simulink model "EngineModel_scaled_15_7_2016_with_new_maps"  (R2021a)
settings: Solver=ode4  StartTime=0.0  StopTime=30  FixedStep=0.2  RelTol=1e-3  EnableMultiTasking=on
values from neighbouring files (symbols this model uses):
  Fanmap_2 = [1 1 1 1 1 1 1 1 1 1 275.724 325.4224 ... (330 elements, 10x3x11)]    [enginemaps2.mat]
  HPCompmap_2 = [1 1 1 1 1 1 1 1 1 1 32.390865 37.6623195 ... (330 elements, 10x3x11)]    [enginemaps2.mat]
  HPTurbinemap_2 = [0.24979968 0.24979968 0.24979968 0.24979968 0.24979968 0.24979968 0.24979968 0.24979968 0.24979968 0.24979968 0.004250667 0.005047667 ... (330 elements, 10x3x11)]    [enginemaps2.mat]
  LPCompmap_2 = [1 1 1 1 1 1 1 1 1 1 34.17260994 40.23277722 ... (330 elements, 10x3x11)]    [enginemaps2.mat]
  LPTurbinemap_2 = [0.665969797 0.665969797 0.665969797 0.665969797 0.665969797 0.665969797 0.665969797 0.665969797 0.00912 0.013173333 0.015706667 0.01672 ... (264 elements, 8x3x11)]    [enginemaps2.mat]
undefined symbols (not defined in the file or in its folder): Adiabatic_compression_fan, Adiabatic_compression_HPC, Adiabatic_compression_LPC, coldnozzle, compression_ram, cond_f2, D, datatables, hotnozzle, HPT1, if_Nth, if_Ntl, if_Z, LPT, performance1, thermo_combustor, turbo
libraries: dspmtrx3 x10, aerolibatmos2 x8, dspsigattribs x3, dspsolvers x2, dspfactors x1
(part 2 of 13)

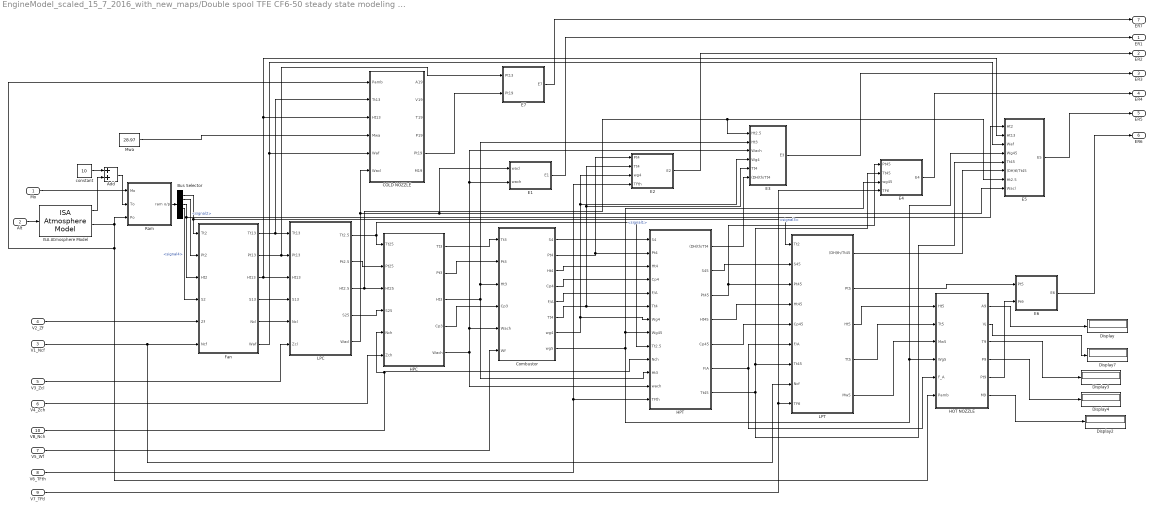
== system EngineModel_scaled_15_7_2016_with_new_maps/Double spool TFE CF6-50 steady state modeling (BOING 747-200)/Error Due to Vs/Error Due To Dv5 ==
  Mo : Inport
  Alt : Inport  Port=2
  V1_Ncf : Inport  Port=3
  V2_Zf : Inport  Port=4
  V3_Zcl : Inport  Port=5
  V4_Zch : Inport  Port=6
  V5_Wf : Inport  Port=7
  V6_TFth : Inport  Port=8
  V7_TFtl : Inport  Port=9
  VB_Nch : Inport  Port=10
  Add : Sum
  Bus Selector : BusSelector  OutputSignals=signal1,signal2,signal3,signal4,signal5
  COLD NOZZLE : Subsystem
  Combustor : Subsystem
  Display{,2..4,7} (5 alike) : Display
  E1 : Subsystem
  E2 : Subsystem
  E3 : Subsystem
  E4 : Subsystem
  E5 : Subsystem
  E6 : Subsystem
  E7 : Subsystem
  Fan : Subsystem
  HOT NOZZLE : Subsystem
  HPC : Subsystem
  HPT : Subsystem
  ISA Atmosphere Model : aerolibatmos2/ISA Atmosphere Model  custom=on  g=9.81  gamma=1.4  R=287  L=0.0065  h_trop=11000  h_strat=20000  rho0=1.225  P0=101325  T0=288  h0=0
  LPC : Subsystem
  LPT : Subsystem
  Mwa : Constant  Value=28.97
  Ram : Subsystem
  constant : Constant  Value=10
  ER1 : Outport
  ER2 : Outport  Port=2
  ER3 : Outport  Port=3
  ER4 : Outport  Port=4
  ER5 : Outport  Port=5
  ER6 : Outport  Port=6
  ER7 : Outport  Port=7
  wires:
  Alt/1 -> ISA Atmosphere Model/1
  Mo/1 -> Ram/1(Mo)
  ISA Atmosphere Model/1 -> Add/2
  Ram/1(ram o/p) -> Bus Selector/1
  ISA Atmosphere Model/3 -> Ram/3(Po), COLD NOZZLE/1(Pamb), HOT NOZZLE/6(Pamb)
  constant/1 -> Add/1
  Add/1 -> Ram/2(To)
  Bus Selector/1 -> Fan/1(Tt2), LPT/1(Tt2)  "<signal1>"
  Bus Selector/2 -> Fan/2(Pt2)  "<signal2>"
  Fan/1(Tt13) -> LPC/1(Tt13), COLD NOZZLE/2(Tt13)
  Fan/2(Pt13) -> E7/1(Pt13), LPC/2(Pt13)
  LPC/1(Tt2.5) -> HPC/1(Tt25), HPT/9(Tt2.5)
  LPC/2(Pt2.5) -> HPC/2(Pt25)
  HPC/1(Tt3) -> Combustor/1(Tt3)
  HPC/2(Pt3) -> Combustor/2(Pt3)
  HPC/3(Ht3) -> Combustor/3(Ht3), E3/2(Ht3), HPT/11(Ht3)
  Combustor/2(Pt4) -> E2/1(Pt4), HPT/2(Pt4)
  Combustor/4(Cp4) -> HPT/4(Cp4)
  Combustor/5(F/A) -> HPT/5(F/A)
  Combustor/6(Tt4) -> E2/2(Tt4), E3/5(Tt4), HPT/6(Tt4)
  LPT/3(Ht5) -> HOT NOZZLE/1(Ht5)
  LPT/4(Tt5) -> HOT NOZZLE/2(Tt5)
  V2_Zf/1 -> Fan/5(Zf)
  V1_Ncf/1 -> LPT/8(Ncf), Fan/6(Ncf)
  V3_Zcl/1 -> LPC/6(Zcl)
  V4_Zch/1 -> HPC/6(Zch)
  VB_Nch/1 -> HPT/10(Nch), HPC/5(Nch)
  V5_Wf/1 -> Combustor/6(Wf)
  V6_TFth/1 -> E2/4(TFth), HPT/13(TFth)
  Combustor/7(wg4) -> E2/3(wg4), E3/4(Wg4), HPT/7(Wg4)
  LPT/5(Mw5) -> HOT NOZZLE/3(Mw5)
  Fan/3(Ht13) -> COLD NOZZLE/3(Ht13), E5/2(Ht13), LPC/3(Ht13)
  Mwa/1 -> COLD NOZZLE/4(Mwa)
  Fan/6(Waf) -> E5/3(Waf), COLD NOZZLE/5(Waf)
  LPC/5(Wacl) -> COLD NOZZLE/6(Wacl), E1/1(wacl), E5/8(Wacl)
  COLD NOZZLE/5(Pt19) -> E7/2(Pt19)
  LPC/3(Ht2.5) -> HPC/3(Ht25), E3/1(Ht2.5), E5/7(Ht2.5)
  LPT/2(Pt5) -> E6/1(Pt5)
  HOT NOZZLE/5(Pt9) -> E6/2(Pt9)
  LPT/1((DH)th/Tt45) -> E5/6((DH)tl/Tt45)
  Combustor/8(wg5) -> E4/3(wg45), HPT/8(Wg45), E5/4(Wg45), HOT NOZZLE/4(Wg5)
  Combustor/3(Ht4) -> HPT/3(Ht4)
  Combustor/1(S4) -> HPT/1(S4)
  HOT NOZZLE/1(A9) -> Display/1
  HOT NOZZLE/2(Vj) -> Display7/1
  HOT NOZZLE/3(T9) -> Display3/1
  HOT NOZZLE/4(P9) -> Display4/1
  HOT NOZZLE/6(M9) -> Display2/1
  Bus Selector/3 -> Fan/3(Ht2), E5/1(Ht2)  "<signal3>"
  Bus Selector/4 -> Fan/4(S2)  "<signal4>"
  Fan/5(Ncl) -> LPC/5(Ncl)
  Fan/4(S13) -> LPC/4(S13)
  LPC/4(S25) -> HPC/4(S25)
  HPC/5(Wach) -> Combustor/5(Wach), E3/3(Wach), E1/2(wach), HPT/12(wach)
  HPT/2(S45) -> LPT/2(S45)
  HPT/3(Pt45) -> E4/1(Pt45), LPT/3(Pt45)
  HPT/4(Ht45) -> LPT/4(Ht45)
  HPT/5(Cp45) -> LPT/5(Cp45)
  HPT/7(Tt45) -> LPT/7(Tt45), E4/2(Tt45), E5/5(Tt45)
  HPT/6(F\A) -> LPT/6(F/A), HOT NOZZLE/5(F_A)
  V7_TFtl/1 -> LPT/9(TFtl), E4/4(TFtl)
  HPT/1((DH)th/Tt4) -> E3/6((DH)th/Tt4)
  E6/1(E6) -> ER6/1
  E5/1(E5) -> ER5/1
  E4/1(E4) -> ER4/1
  E3/1(E3) -> ER3/1
  E2/1(E2) -> ER2/1
  E1/1(E1) -> ER1/1
  E7/1(E7) -> ER7/1
  HPC/4(Cp3) -> Combustor/4(Cp3)

== system EngineModel_scaled_15_7_2016_with_new_maps/Double spool TFE CF6-50 steady state modeling (BOING 747-200)/Error Due to Vs/Error Due To Dv6 ==
  Mo : Inport
  Alt : Inport  Port=2
  V1_Ncf : Inport  Port=3
  V2_Zf : Inport  Port=4
  V3_Zcl : Inport  Port=5
  V4_Zch : Inport  Port=6
  V5_Wf : Inport  Port=7
  V6_TFth : Inport  Port=8
  V7_TFtl : Inport  Port=9
  VB_Nch : Inport  Port=10
  Add : Sum
  Bus Selector : BusSelector  OutputSignals=signal1,signal2,signal3,signal4,signal5
  COLD NOZZLE : Subsystem
  Combustor : Subsystem
  Display{,2..4,7} (5 alike) : Display
  E1 : Subsystem
  E2 : Subsystem
  E3 : Subsystem
  E4 : Subsystem
  E5 : Subsystem
  E6 : Subsystem
  E7 : Subsystem
  Fan : Subsystem
  HOT NOZZLE : Subsystem
  HPC : Subsystem
  HPT : Subsystem
  ISA Atmosphere Model : aerolibatmos2/ISA Atmosphere Model  custom=on  g=9.81  gamma=1.4  R=287  L=0.0065  h_trop=11000  h_strat=20000  rho0=1.225  P0=101325  T0=288  h0=0
  LPC : Subsystem
  LPT : Subsystem
  Mwa : Constant  Value=28.97
  Ram : Subsystem
  constant : Constant  Value=10
  ER1 : Outport
  ER2 : Outport  Port=2
  ER3 : Outport  Port=3
  ER4 : Outport  Port=4
  ER5 : Outport  Port=5
  ER6 : Outport  Port=6
  ER7 : Outport  Port=7
  wires:
  HPC/4(Cp3) -> Combustor/4(Cp3)
  E7/1(E7) -> ER7/1
  E1/1(E1) -> ER1/1
  E2/1(E2) -> ER2/1
  E3/1(E3) -> ER3/1
  E4/1(E4) -> ER4/1
  E5/1(E5) -> ER5/1
  E6/1(E6) -> ER6/1
  HPT/1((DH)th/Tt4) -> E3/6((DH)th/Tt4)
  V7_TFtl/1 -> E4/4(TFtl), LPT/9(TFtl)
  HPT/6(F\A) -> HOT NOZZLE/5(F_A), LPT/6(F/A)
  HPT/7(Tt45) -> E5/5(Tt45), E4/2(Tt45), LPT/7(Tt45)
  HPT/5(Cp45) -> LPT/5(Cp45)
  HPT/4(Ht45) -> LPT/4(Ht45)
  HPT/3(Pt45) -> LPT/3(Pt45), E4/1(Pt45)
  HPT/2(S45) -> LPT/2(S45)
  HPC/5(Wach) -> HPT/12(wach), E1/2(wach), E3/3(Wach), Combustor/5(Wach)
  LPC/4(S25) -> HPC/4(S25)
  Fan/4(S13) -> LPC/4(S13)
  Fan/5(Ncl) -> LPC/5(Ncl)
  Bus Selector/4 -> Fan/4(S2)  "<signal4>"
  Bus Selector/3 -> E5/1(Ht2), Fan/3(Ht2)  "<signal3>"
  HOT NOZZLE/6(M9) -> Display2/1
  HOT NOZZLE/4(P9) -> Display4/1
  HOT NOZZLE/3(T9) -> Display3/1
  HOT NOZZLE/2(Vj) -> Display7/1
  HOT NOZZLE/1(A9) -> Display/1
  Combustor/1(S4) -> HPT/1(S4)
  Combustor/3(Ht4) -> HPT/3(Ht4)
  Combustor/8(wg5) -> HOT NOZZLE/4(Wg5), E5/4(Wg45), HPT/8(Wg45), E4/3(wg45)
  LPT/1((DH)th/Tt45) -> E5/6((DH)tl/Tt45)
  HOT NOZZLE/5(Pt9) -> E6/2(Pt9)
  LPT/2(Pt5) -> E6/1(Pt5)
  LPC/3(Ht2.5) -> E5/7(Ht2.5), E3/1(Ht2.5), HPC/3(Ht25)
  COLD NOZZLE/5(Pt19) -> E7/2(Pt19)
  LPC/5(Wacl) -> E5/8(Wacl), E1/1(wacl), COLD NOZZLE/6(Wacl)
  Fan/6(Waf) -> COLD NOZZLE/5(Waf), E5/3(Waf)
  Mwa/1 -> COLD NOZZLE/4(Mwa)
  Fan/3(Ht13) -> LPC/3(Ht13), E5/2(Ht13), COLD NOZZLE/3(Ht13)
  LPT/5(Mw5) -> HOT NOZZLE/3(Mw5)
  Combustor/7(wg4) -> HPT/7(Wg4), E3/4(Wg4), E2/3(wg4)
  V6_TFth/1 -> HPT/13(TFth), E2/4(TFth)
  V5_Wf/1 -> Combustor/6(Wf)
  VB_Nch/1 -> HPC/5(Nch), HPT/10(Nch)
  V4_Zch/1 -> HPC/6(Zch)
  V3_Zcl/1 -> LPC/6(Zcl)
  V1_Ncf/1 -> Fan/6(Ncf), LPT/8(Ncf)
  V2_Zf/1 -> Fan/5(Zf)
  LPT/4(Tt5) -> HOT NOZZLE/2(Tt5)
  LPT/3(Ht5) -> HOT NOZZLE/1(Ht5)
  Combustor/6(Tt4) -> HPT/6(Tt4), E3/5(Tt4), E2/2(Tt4)
  Combustor/5(F/A) -> HPT/5(F/A)
  Combustor/4(Cp4) -> HPT/4(Cp4)
  Combustor/2(Pt4) -> HPT/2(Pt4), E2/1(Pt4)
  HPC/3(Ht3) -> HPT/11(Ht3), E3/2(Ht3), Combustor/3(Ht3)
  HPC/2(Pt3) -> Combustor/2(Pt3)
  HPC/1(Tt3) -> Combustor/1(Tt3)
  LPC/2(Pt2.5) -> HPC/2(Pt25)
  LPC/1(Tt2.5) -> HPT/9(Tt2.5), HPC/1(Tt25)
  Fan/2(Pt13) -> LPC/2(Pt13), E7/1(Pt13)
  Fan/1(Tt13) -> COLD NOZZLE/2(Tt13), LPC/1(Tt13)
  Bus Selector/2 -> Fan/2(Pt2)  "<signal2>"
  Bus Selector/1 -> LPT/1(Tt2), Fan/1(Tt2)  "<signal1>"
  Add/1 -> Ram/2(To)
  constant/1 -> Add/1
  ISA Atmosphere Model/3 -> HOT NOZZLE/6(Pamb), COLD NOZZLE/1(Pamb), Ram/3(Po)
  Ram/1(ram o/p) -> Bus Selector/1
  ISA Atmosphere Model/1 -> Add/2
  Mo/1 -> Ram/1(Mo)
  Alt/1 -> ISA Atmosphere Model/1

== system EngineModel_scaled_15_7_2016_with_new_maps/Double spool TFE CF6-50 steady state modeling (BOING 747-200)/Error Due to Vs/Error Due To Dv7 ==
  Mo : Inport
  Alt : Inport  Port=2
  V1_Ncf : Inport  Port=3
  V2_Zf : Inport  Port=4
  V3_Zcl : Inport  Port=5
  V4_Zch : Inport  Port=6
  V5_Wf : Inport  Port=7
  V6_TFth : Inport  Port=8
  V7_TFtl : Inport  Port=9
  VB_Nch : Inport  Port=10
  Add : Sum
  Bus Selector : BusSelector  OutputSignals=signal1,signal2,signal3,signal4,signal5
  COLD NOZZLE : Subsystem
  Combustor : Subsystem
  Display{,2..4,7} (5 alike) : Display
  E1 : Subsystem
  E2 : Subsystem
  E3 : Subsystem
  E4 : Subsystem
  E5 : Subsystem
  E6 : Subsystem
  E7 : Subsystem
  Fan : Subsystem
  HOT NOZZLE : Subsystem
  HPC : Subsystem
  HPT : Subsystem
  ISA Atmosphere Model : aerolibatmos2/ISA Atmosphere Model  custom=on  g=9.81  gamma=1.4  R=287  L=0.0065  h_trop=11000  h_strat=20000  rho0=1.225  P0=101325  T0=288  h0=0
  LPC : Subsystem
  LPT : Subsystem
  Mwa : Constant  Value=28.97
  Ram : Subsystem
  constant : Constant  Value=10
  ER1 : Outport
  ER2 : Outport  Port=2
  ER3 : Outport  Port=3
  ER4 : Outport  Port=4
  ER5 : Outport  Port=5
  ER6 : Outport  Port=6
  ER7 : Outport  Port=7
  wires:
  Alt/1 -> ISA Atmosphere Model/1
  Mo/1 -> Ram/1(Mo)
  ISA Atmosphere Model/1 -> Add/2
  Ram/1(ram o/p) -> Bus Selector/1
  ISA Atmosphere Model/3 -> Ram/3(Po), COLD NOZZLE/1(Pamb), HOT NOZZLE/6(Pamb)
  constant/1 -> Add/1
  Add/1 -> Ram/2(To)
  Bus Selector/1 -> Fan/1(Tt2), LPT/1(Tt2)  "<signal1>"
  Bus Selector/2 -> Fan/2(Pt2)  "<signal2>"
  Fan/1(Tt13) -> LPC/1(Tt13), COLD NOZZLE/2(Tt13)
  Fan/2(Pt13) -> E7/1(Pt13), LPC/2(Pt13)
  LPC/1(Tt2.5) -> HPC/1(Tt25), HPT/9(Tt2.5)
  LPC/2(Pt2.5) -> HPC/2(Pt25)
  HPC/1(Tt3) -> Combustor/1(Tt3)
  HPC/2(Pt3) -> Combustor/2(Pt3)
  HPC/3(Ht3) -> Combustor/3(Ht3), E3/2(Ht3), HPT/11(Ht3)
  Combustor/2(Pt4) -> E2/1(Pt4), HPT/2(Pt4)
  Combustor/4(Cp4) -> HPT/4(Cp4)
  Combustor/5(F/A) -> HPT/5(F/A)
  Combustor/6(Tt4) -> E2/2(Tt4), E3/5(Tt4), HPT/6(Tt4)
  LPT/3(Ht5) -> HOT NOZZLE/1(Ht5)
  LPT/4(Tt5) -> HOT NOZZLE/2(Tt5)
  V2_Zf/1 -> Fan/5(Zf)
  V1_Ncf/1 -> LPT/8(Ncf), Fan/6(Ncf)
  V3_Zcl/1 -> LPC/6(Zcl)
  V4_Zch/1 -> HPC/6(Zch)
  VB_Nch/1 -> HPT/10(Nch), HPC/5(Nch)
  V5_Wf/1 -> Combustor/6(Wf)
  V6_TFth/1 -> E2/4(TFth), HPT/13(TFth)
  Combustor/7(wg4) -> E2/3(wg4), E3/4(Wg4), HPT/7(Wg4)
  LPT/5(Mw5) -> HOT NOZZLE/3(Mw5)
  Fan/3(Ht13) -> COLD NOZZLE/3(Ht13), E5/2(Ht13), LPC/3(Ht13)
  Mwa/1 -> COLD NOZZLE/4(Mwa)
  Fan/6(Waf) -> E5/3(Waf), COLD NOZZLE/5(Waf)
  LPC/5(Wacl) -> COLD NOZZLE/6(Wacl), E1/1(wacl), E5/8(Wacl)
  COLD NOZZLE/5(Pt19) -> E7/2(Pt19)
  LPC/3(Ht2.5) -> HPC/3(Ht25), E3/1(Ht2.5), E5/7(Ht2.5)
  LPT/2(Pt5) -> E6/1(Pt5)
  HOT NOZZLE/5(Pt9) -> E6/2(Pt9)
  LPT/1((DH)th/Tt45) -> E5/6((DH)tl/Tt45)
  Combustor/8(wg5) -> E4/3(wg45), HPT/8(Wg45), E5/4(Wg45), HOT NOZZLE/4(Wg5)
  Combustor/3(Ht4) -> HPT/3(Ht4)
  Combustor/1(S4) -> HPT/1(S4)
  HOT NOZZLE/1(A9) -> Display/1
  HOT NOZZLE/2(Vj) -> Display7/1
  HOT NOZZLE/3(T9) -> Display3/1
  HOT NOZZLE/4(P9) -> Display4/1
  HOT NOZZLE/6(M9) -> Display2/1
  Bus Selector/3 -> Fan/3(Ht2), E5/1(Ht2)  "<signal3>"
  Bus Selector/4 -> Fan/4(S2)  "<signal4>"
  Fan/5(Ncl) -> LPC/5(Ncl)
  Fan/4(S13) -> LPC/4(S13)
  LPC/4(S25) -> HPC/4(S25)
  HPC/5(Wach) -> Combustor/5(Wach), E3/3(Wach), E1/2(wach), HPT/12(wach)
  HPT/2(S45) -> LPT/2(S45)
  HPT/3(Pt45) -> E4/1(Pt45), LPT/3(Pt45)
  HPT/4(Ht45) -> LPT/4(Ht45)
  HPT/5(Cp45) -> LPT/5(Cp45)
  HPT/7(Tt45) -> LPT/7(Tt45), E4/2(Tt45), E5/5(Tt45)
  HPT/6(F\A) -> LPT/6(F/A), HOT NOZZLE/5(F_A)
  V7_TFtl/1 -> LPT/9(TFtl), E4/4(TFtl)
  HPT/1((DH)th/Tt4) -> E3/6((DH)th/Tt4)
  E6/1(E6) -> ER6/1
  E5/1(E5) -> ER5/1
  E4/1(E4) -> ER4/1
  E3/1(E3) -> ER3/1
  E2/1(E2) -> ER2/1
  E1/1(E1) -> ER1/1
  E7/1(E7) -> ER7/1
  HPC/4(Cp3) -> Combustor/4(Cp3)

== system EngineModel_scaled_15_7_2016_with_new_maps/Double spool TFE CF6-50 steady state modeling (BOING 747-200)/Off- Design Module/COLD NOZZLE ==
  Po : Inport
  Tt13 : Inport  Port=2
  Ht13 : Inport  Port=3
  Mwa : Inport  Port=4
  Waf : Inport  Port=5
  Wacl : Inport  Port=6
  Demux : Demux  Outputs=6
      settings: DisplayOption=none
  Display : Display
  Display1 : Display
  Interpreted MATLAB Function : MATLABFcn  MATLABFcn=coldnozzle(u(1),u(2),u(3),u(4),u(5),u(6))  OutputDimensions=6
  Mux : Mux  Inputs=6
      settings: DisplayOption=signals
  A19 : Outport
  V19 : Outport  Port=2
  T19 : Outport  Port=3
  P19 : Outport  Port=4
  Pt19 : Outport  Port=5
  M19 : Outport  Port=6
  wires:
  Mux/1 -> Interpreted MATLAB Function/1
  Interpreted MATLAB Function/1 -> Demux/1
  Ht13/1 -> Mux/3
  Mwa/1 -> Mux/4
  Waf/1 -> Mux/5
  Wacl/1 -> Mux/6
  Demux/1 -> A19/1
  Demux/2 -> Display/1, V19/1
  Demux/3 -> Display1/1, T19/1
  Demux/4 -> P19/1
  Demux/5 -> Pt19/1
  Demux/6 -> M19/1
  Tt13/1 -> Mux/2
  Po/1 -> Mux/1

== system EngineModel_scaled_15_7_2016_with_new_maps/Double spool TFE CF6-50 steady state modeling (BOING 747-200)/Off- Design Module/Combustor ==
  Tt3 : Inport
  Pt3 : Inport  Port=2
  Ht3 : Inport  Port=3
  Cp3 : Inport  Port=4
  Wach : Inport  Port=5
  Wf : Inport  Port=6
  (1-percent bleed airpcwb2) : Constant  Value=0.9
  Add1 : Sum
  Add2 : Sum
  Display{1..2,4..7} (6 alike) : Display
  Product : Product
  Thermo_combustor : Subsystem  TreatAsAtomicUnit=on
  combustor o/p enthalpy : Subsystem  TreatAsAtomicUnit=on
  combustor o/p pressure : Subsystem
  S4 : Outport
  Pt4 : Outport  Port=2
  Ht4 : Outport  Port=3
  Cp4 : Outport  Port=4
  F/A : Outport  Port=5
  Tt4 : Outport  Port=6
  wg4 : Outport  Port=7
  wg5 : Outport  Port=8
  wires:
  Pt3/1 -> combustor o/p pressure/1(Pt3)
  Tt3/1 -> combustor o/p pressure/2(Tt3)
  Wf/1 -> Add1/2, Add2/2, combustor o/p enthalpy/1("wf ")
  Ht3/1 -> combustor o/p enthalpy/3(Ht3)
  combustor o/p pressure/1(Pt4) -> Display1/1, Pt4/1, Thermo_combustor/1(Pt4)
  combustor o/p enthalpy/2(F_A) -> F/A/1, Thermo_combustor/4(F/A)
  Thermo_combustor/2(S4) -> Display7/1, S4/1
  Thermo_combustor/3(Cp4) -> Cp4/1
  Thermo_combustor/1(Tt4) -> Tt4/1, Display4/1
  Add1/1 -> Display2/1, wg5/1
  Wach/1 -> Product/2, combustor o/p pressure/3(wach), combustor o/p enthalpy/2(wach), Add1/1
  combustor o/p enthalpy/1(Ht4) -> Ht4/1, Display5/1, Thermo_combustor/3("Ht4 ")
  Product/1 -> Add2/1
  (1-percent bleed airpcwb2)/1 -> Product/1
  Add2/1 -> Display6/1, combustor o/p enthalpy/4(wg4), wg4/1
  Cp3/1 -> Thermo_combustor/2(Cp3)

== system EngineModel_scaled_15_7_2016_with_new_maps/Double spool TFE CF6-50 steady state modeling (BOING 747-200)/Off- Design Module/E1 ==
  wacl : Inport
  wach : Inport  Port=2
  Abs : Abs
  Data Type Conversion : DataTypeConversion  OutDataTypeStr=boolean
  Display : Display
  Divide1 : Product  Inputs=*/
  Sum : Sum  Inputs=-+  SaturateOnIntegerOverflow=on
  condition : Subsystem
  E1 : Outport
  cond1 : Outport  Port=2  OutDataTypeStr=boolean
  wires:
  wacl/1 -> Sum/1
  wach/1 -> Divide1/2, Sum/2
  Sum/1 -> Divide1/1
  Abs/1 -> condition/1(In1)
  Data Type Conversion/1 -> cond1/1
  condition/1(Out1) -> Data Type Conversion/1
  Divide1/1 -> Display/1, Abs/1, E1/1

== system EngineModel_scaled_15_7_2016_with_new_maps/Double spool TFE CF6-50 steady state modeling (BOING 747-200)/Off- Design Module/E2 ==
  Pt4 : Inport
  Tt4 : Inport  Port=2
  wg4 : Inport  Port=3
  TFth : Inport  Port=4
  Abs : Abs
  Constant : Constant  Value=100000
  Data Type Conversion : DataTypeConversion  OutDataTypeStr=boolean
  Display{,1..4} (5 alike) : Display
  Divide1 : Product  Inputs=/*
  Divide2 : Product  Inputs=/*
  Divide3 : Product  Inputs=/*
  Product5 : Product  Inputs=**  SaturateOnIntegerOverflow=on  OutDataTypeStr=Inherit: Same as first input
  Sqrt1 : Sqrt  SaturateOnIntegerOverflow=on
  Sum : Sum  Inputs=+-  SaturateOnIntegerOverflow=on
  condition : Subsystem
  E2 : Outport
  cond2 : Outport  Port=2  OutDataTypeStr=boolean
  wires:
  Sum/1 -> Divide1/2
  TFth/1 -> Display1/1, Sum/2
  Divide2/1 -> Sum/1, Display2/1, Divide1/1
  Tt4/1 -> Sqrt1/1
  wg4/1 -> Display3/1, Product5/2
  Sqrt1/1 -> Product5/1
  Product5/1 -> Divide2/2
  Pt4/1 -> Divide3/2
  Constant/1 -> Divide3/1
  Divide3/1 -> Divide2/1, Display4/1
  Abs/1 -> condition/1(In1)
  Data Type Conversion/1 -> cond2/1
  condition/1(Out1) -> Data Type Conversion/1
  Divide1/1 -> Abs/1, E2/1, Display/1

== system EngineModel_scaled_15_7_2016_with_new_maps/Double spool TFE CF6-50 steady state modeling (BOING 747-200)/Off- Design Module/E3 ==
  Ht2.5 : Inport
  Ht3 : Inport  Port=2
  Wach : Inport  Port=3
  Wg4 : Inport  Port=4
  Tt4 : Inport  Port=5
  (DH)th/Tt4 : Inport  Port=6
  Abs : Abs
  Constant : Constant  Value=4.184
  Data Type Conversion : DataTypeConversion  OutDataTypeStr=boolean
  Display1 : Display
  Display2 : Display
  Divide1 : Product  Inputs=/*
  Divide2 : Product  Inputs=/*
  Divide3 : Product  Inputs=/*
  Product1 : Product  Inputs=**  SaturateOnIntegerOverflow=on  OutDataTypeStr=Inherit: Same as first input
  Product2 : Product  Inputs=**  SaturateOnIntegerOverflow=on  OutDataTypeStr=Inherit: Same as first input
  Sum : Sum  Inputs=+-  SaturateOnIntegerOverflow=on
  Sum1 : Sum  Inputs=+-  SaturateOnIntegerOverflow=on
  condition : Subsystem
  E3 : Outport
  cond3 : Outport  Port=2  OutDataTypeStr=boolean
  wires:
  Ht2.5/1 -> Sum/2
  Ht3/1 -> Sum/1
  Sum/1 -> Product1/2
  Wach/1 -> Product1/1
  Wg4/1 -> Product2/1
  Tt4/1 -> Product2/2
  Product2/1 -> Divide1/1
  Divide1/1 -> Sum1/1, Divide2/1, Display1/1
  Sum1/1 -> Divide2/2
  Product1/1 -> Divide3/2
  Divide3/1 -> Divide1/2
  Constant/1 -> Divide3/1
  (DH)th/Tt4/1 -> Sum1/2
  Abs/1 -> condition/1(In1)
  Data Type Conversion/1 -> cond3/1
  condition/1(Out1) -> Data Type Conversion/1
  Divide2/1 -> Abs/1, E3/1, Display2/1

== system EngineModel_scaled_15_7_2016_with_new_maps/Double spool TFE CF6-50 steady state modeling (BOING 747-200)/Off- Design Module/E4 ==
  Pt45 : Inport
  Tt45 : Inport  Port=2
  wg45 : Inport  Port=3
  TFtl : Inport  Port=4
  Abs : Abs
  Constant : Constant  Value=100000
  Data Type Conversion : DataTypeConversion  OutDataTypeStr=boolean
  Display : Display
  Display1 : Display
  Divide1 : Product  Inputs=/*
  Divide2 : Product  Inputs=/*
  Divide3 : Product  Inputs=/*
  Product5 : Product  Inputs=**  SaturateOnIntegerOverflow=on  OutDataTypeStr=Inherit: Same as first input
  Sqrt1 : Sqrt  SaturateOnIntegerOverflow=on
  Sum : Sum  Inputs=+-  SaturateOnIntegerOverflow=on
  condition : Subsystem
  E4 : Outport
  cond4 : Outport  Port=2  OutDataTypeStr=boolean
  wires:
  Product5/1 -> Divide2/2
  Sqrt1/1 -> Product5/1
  wg45/1 -> Product5/2
  Tt45/1 -> Sqrt1/1
  Divide2/1 -> Sum/1, Divide1/1, Display1/1
  TFtl/1 -> Sum/2
  Sum/1 -> Divide1/2
  Pt45/1 -> Divide3/2
  Constant/1 -> Divide3/1
  Divide3/1 -> Divide2/1
  Abs/1 -> condition/1(In1)
  Data Type Conversion/1 -> cond4/1
  condition/1(Out1) -> Data Type Conversion/1
  Divide1/1 -> Abs/1, E4/1, Display/1

== system EngineModel_scaled_15_7_2016_with_new_maps/Double spool TFE CF6-50 steady state modeling (BOING 747-200)/Off- Design Module/E5 ==
  Ht2 : Inport
  Ht13 : Inport  Port=2
  Waf : Inport  Port=3
  Wg45 : Inport  Port=4
  Tt45 : Inport  Port=5
  (DH)tl/Tt45 : Inport  Port=6
  Ht2.5 : Inport  Port=7
  Wacl : Inport  Port=8
  Abs : Abs
  Constant : Constant  Value=4.184
  Data Type Conversion : DataTypeConversion  OutDataTypeStr=boolean
  Display : Display
  Display1 : Display
  Display3 : Display
  Divide1 : Product  Inputs=/*
  Divide2 : Product  Inputs=/*
  Divide3 : Product  Inputs=/*
  Product1 : Product  Inputs=**  SaturateOnIntegerOverflow=on  OutDataTypeStr=Inherit: Same as first input
  Product2 : Product  Inputs=**  SaturateOnIntegerOverflow=on  OutDataTypeStr=Inherit: Same as first input
  Product4 : Product  Inputs=**  SaturateOnIntegerOverflow=on  OutDataTypeStr=Inherit: Same as first input
  Sum : Sum  Inputs=+-  SaturateOnIntegerOverflow=on
  Sum1 : Sum  Inputs=+-  SaturateOnIntegerOverflow=on
  Sum2 : Sum  Inputs=+-  SaturateOnIntegerOverflow=on
  Sum3 : Sum  SaturateOnIntegerOverflow=on
  condition : Subsystem
  E5 : Outport
  cond5 : Outport  Port=2  OutDataTypeStr=boolean
  wires:
  (DH)tl/Tt45/1 -> Sum1/2
  Sum1/1 -> Divide2/2
  Divide1/1 -> Sum1/1, Display1/1, Divide2/1
  Product2/1 -> Divide1/1
  Tt45/1 -> Product2/2
  Wg45/1 -> Product2/1
  Waf/1 -> Product1/1
  Sum/1 -> Product1/2
  Ht2/1 -> Sum/2
  Wacl/1 -> Product4/1
  Sum2/1 -> Product4/2
  Ht2.5/1 -> Sum2/1
  Ht13/1 -> Sum2/2, Sum/1
  Product4/1 -> Sum3/1
  Product1/1 -> Sum3/2
  Sum3/1 -> Divide3/2
  Constant/1 -> Divide3/1
  Divide3/1 -> Divide1/2
  Abs/1 -> condition/1(In1)
  Data Type Conversion/1 -> cond5/1
  condition/1(Out1) -> Data Type Conversion/1
  Divide2/1 -> Abs/1, E5/1, Display/1

== system EngineModel_scaled_15_7_2016_with_new_maps/Double spool TFE CF6-50 steady state modeling (BOING 747-200)/Off- Design Module/E6 ==
  Pt5 : Inport
  Pt9 : Inport  Port=2
  Abs : Abs
  Data Type Conversion : DataTypeConversion  OutDataTypeStr=boolean
  Display{,1..4} (5 alike) : Display
  Divide1 : Product  Inputs=/*
  Sum : Sum  Inputs=+-  SaturateOnIntegerOverflow=on
  condition : Subsystem
  E6 : Outport
  cond6 : Outport  Port=2  OutDataTypeStr=boolean
  wires:
  Sum/1 -> Divide1/2
  Pt5/1 -> Display2/1, Sum/2
  Pt9/1 -> Display1/1, Divide1/1, Sum/1
  Abs/1 -> condition/1(In1)
  Data Type Conversion/1 -> Display4/1, cond6/1
  condition/1(Out1) -> Display3/1, Data Type Conversion/1
  Divide1/1 -> Abs/1, E6/1, Display/1

== system EngineModel_scaled_15_7_2016_with_new_maps/Double spool TFE CF6-50 steady state modeling (BOING 747-200)/Off- Design Module/E7 ==
  Pt13 : Inport
  Pt19 : Inport  Port=2
  Abs : Abs
  Data Type Conversion : DataTypeConversion  OutDataTypeStr=boolean
  Display : Display
  Divide1 : Product  Inputs=/*
  Sum : Sum  Inputs=+-  SaturateOnIntegerOverflow=on
  condition : Subsystem
  E7 : Outport
  "cond7 " : Outport  Port=2  OutDataTypeStr=boolean
  wires:
  Sum/1 -> Divide1/2
  Pt13/1 -> Sum/2
  Pt19/1 -> Divide1/1, Sum/1
  Abs/1 -> condition/1(In1)
  Data Type Conversion/1 -> "cond7 "/1
  condition/1(Out1) -> Data Type Conversion/1
  Divide1/1 -> Abs/1, E7/1, Display/1

== system EngineModel_scaled_15_7_2016_with_new_maps/Double spool TFE CF6-50 steady state modeling (BOING 747-200)/Off- Design Module/Fan ==
  Tt2 : Inport
  Pt2 : Inport  Port=2
  Ht2 : Inport  Port=3
  S2 : Inport  Port=4
  Zf : Inport  Port=5
  Ncf : Inport  Port=6
  (Po)Ref : Constant  Value=101325
  (To)Ref : Constant  Value=288
  (To)Ref1 : Constant  Value=288
  (To)Ref2 : Constant  Value=288
  Adiabatic compression : Subsystem
  Display{1..7} (7 alike) : Display
  Fan Map : Subsystem
  Product{1..3,6..7} (5 alike) : Product  Inputs=*/  SaturateOnIntegerOverflow=on  OutDataTypeStr=Inherit: Same as first input
  Product10 : Product  Inputs=**  SaturateOnIntegerOverflow=on  OutDataTypeStr=Inherit: Same as first input
  Product4 : Product  Inputs=**  SaturateOnIntegerOverflow=on  OutDataTypeStr=Inherit: Same as first input
  Product5 : Product  Inputs=/*  SaturateOnIntegerOverflow=on  OutDataTypeStr=Inherit: Same as first input
  Product8 : Product  Inputs=/*  SaturateOnIntegerOverflow=on  OutDataTypeStr=Inherit: Same as first input
  Product9 : Product  Inputs=/*  SaturateOnIntegerOverflow=on  OutDataTypeStr=Inherit: Same as first input
  Sqrt1 : Sqrt  SaturateOnIntegerOverflow=on
  Sqrt2 : Sqrt  SaturateOnIntegerOverflow=on
  Sqrt4 : Sqrt  SaturateOnIntegerOverflow=on
  theta13D : Constant  Value=1.04266
  theta2D : Constant  Value=0.9532186
  Tt13 : Outport
  Pt13 : Outport  Port=2
  Ht13 : Outport  Port=3
  S13 : Outport  Port=4
  Ncl : Outport  Port=5
  Waf : Outport  Port=6
  wires:
  Zf/1 -> Fan Map/1(Zf)
  Fan Map/1(Prf) -> Adiabatic compression/3(Prf)
  Fan Map/2(etaf) -> Adiabatic compression/4(etaf)
  Pt2/1 -> Product3/1, Adiabatic compression/2(Pt2), Display3/1
  Tt2/1 -> Product6/1, Adiabatic compression/1(Tt2), Product1/1
  Adiabatic compression/1(Tt13) -> Display1/1, Product7/1, Tt13/1
  Adiabatic compression/3(Ht13) -> Display5/1, Ht13/1
  Product4/1 -> Display4/1, Ncl/1
  (To)Ref1/1 -> Product7/2
  Product7/1 -> Sqrt1/1
  Sqrt1/1 -> Product8/2
  theta13D/1 -> Product8/1
  theta2D/1 -> Product9/1
  Product8/1 -> Product2/1
  Product9/1 -> Product2/2
  (To)Ref2/1 -> Product6/2
  Ncf/1 -> Product4/2, Fan Map/2(Ncf)
  Product6/1 -> Sqrt2/1
  Sqrt2/1 -> Product9/2
  Product2/1 -> Product4/1
  Product1/1 -> Sqrt4/1
  (To)Ref/1 -> Product1/2
  (Po)Ref/1 -> Product3/2
  Product3/1 -> Product5/2
  Sqrt4/1 -> Product5/1
  Fan Map/3(MFPf) -> Product10/2
  Product5/1 -> Product10/1
  Product10/1 -> Display7/1, Waf/1
  Ht2/1 -> Adiabatic compression/5(Ht2)
  S2/1 -> Adiabatic compression/6(S2)
  Adiabatic compression/2(Pt13) -> Display2/1, Pt13/1
  Adiabatic compression/4(S13) -> Display6/1, S13/1

== system EngineModel_scaled_15_7_2016_with_new_maps/Double spool TFE CF6-50 steady state modeling (BOING 747-200)/Off- Design Module/HOT NOZZLE ==
  Ht5 : Inport
  Tt5 : Inport  Port=2
  Mw5 : Inport  Port=3
  Wg5 : Inport  Port=4
  F_A : Inport  Port=5
  Pamb : Inport  Port=6
  Demux : Demux  Outputs=6
      settings: DisplayOption=none
  Display : Display
  Interpreted MATLAB Function : MATLABFcn  MATLABFcn=hotnozzle(u(1),u(2),u(3),u(4),u(5),u(6))  OutputDimensions=6
  Mux : Mux  Inputs=6
      settings: DisplayOption=signals
  A9 : Outport
  Vj : Outport  Port=2
  T9 : Outport  Port=3
  P9 : Outport  Port=4
  Pt9 : Outport  Port=5
  M9 : Outport  Port=6
  wires:
  Mux/1 -> Interpreted MATLAB Function/1
  Interpreted MATLAB Function/1 -> Demux/1
  Ht5/1 -> Mux/3
  Mw5/1 -> Mux/4
  Wg5/1 -> Mux/5
  F_A/1 -> Mux/6
  Demux/1 -> A9/1
  Demux/2 -> Display/1, Vj/1
  Demux/3 -> T9/1
  Demux/4 -> P9/1
  Demux/5 -> Pt9/1
  Demux/6 -> M9/1
  Tt5/1 -> Mux/2
  Pamb/1 -> Mux/1

== system EngineModel_scaled_15_7_2016_with_new_maps/Double spool TFE CF6-50 steady state modeling (BOING 747-200)/Off- Design Module/HPC ==
  Tt25 : Inport
  Pt25 : Inport  Port=2
  Ht25 : Inport  Port=3
  S25 : Inport  Port=4
  Nch : Inport  Port=5
  Zch : Inport  Port=6
  (Po)Ref : Constant  Value=101325
  (To)Ref : Constant  Value=288
  Adiabatic compression : Subsystem
  Display{,1..4} (5 alike) : Display
  HPC Map : Subsystem
  Product2 : Product  Inputs=*/  SaturateOnIntegerOverflow=on  OutDataTypeStr=Inherit: Same as first input
  Product4 : Product  Inputs=*/  SaturateOnIntegerOverflow=on  OutDataTypeStr=Inherit: Same as first input
  Product5 : Product  Inputs=/*  SaturateOnIntegerOverflow=on  OutDataTypeStr=Inherit: Same as first input
  Product6 : Product  Inputs=**  SaturateOnIntegerOverflow=on  OutDataTypeStr=Inherit: Same as first input
  Sqrt1 : Sqrt  SaturateOnIntegerOverflow=on
  To File : ToFile  Filename=datatable2.mat  MatrixName=bes2
  Tt3 : Outport
  Pt3 : Outport  Port=2
  Ht3 : Outport  Port=3
  Cp3 : Outport  Port=4
  Wach : Outport  Port=5
  MFPch : Outport  Port=6
  wires:
  Zch/1 -> HPC Map/1(Zch)
  Nch/1 -> HPC Map/2(Nch)
  Tt25/1 -> Adiabatic compression/1(Tt25), Product4/1
  Pt25/1 -> Adiabatic compression/2(Pt25), Product2/1
  HPC Map/2(etach) -> Adiabatic compression/4(etach)
  (Po)Ref/1 -> Product2/2
  (To)Ref/1 -> Product4/2
  Adiabatic compression/1(Tt3) -> Display1/1, Tt3/1
  Adiabatic compression/2(Pt3) -> Display4/1, Pt3/1
  Adiabatic compression/3(Ht3) -> Display/1, Ht3/1
  Ht25/1 -> Adiabatic compression/5(Ht25)
  S25/1 -> Adiabatic compression/6(S25)
  Adiabatic compression/4(S3) -> Display3/1
  ? -> ?
  ? -> ?
  Sqrt1/1 -> Product5/1
  Product6/1 -> Product5/2
  Product5/1 -> Display2/1, Wach/1
  HPC Map/3(MFPch) -> MFPch/1, Product6/2
  Product4/1 -> Sqrt1/1
  Product2/1 -> Product6/1
  Adiabatic compression/5(Cp3) -> Cp3/1
  HPC Map/1(Prch) -> To File/1, Adiabatic compression/3(Prch)

== system EngineModel_scaled_15_7_2016_with_new_maps/Double spool TFE CF6-50 steady state modeling (BOING 747-200)/Off- Design Module/HPT ==
  S4 : Inport
  Pt4 : Inport  Port=2
  Ht4 : Inport  Port=3
  Cp4 : Inport  Port=4
  F/A : Inport  Port=5
  Tt4 : Inport  Port=6
  Wg4 : Inport  Port=7
  Wg45 : Inport  Port=8
  Tt2.5 : Inport  Port=9
  Nch : Inport  Port=10
  Ht3 : Inport  Port=11
  wach : Inport  Port=12
  TFth : Inport  Port=13
  " \"F/At= 0.9 * F/Acch\"" : Constant  Value=0.9
  " HP turbine" : Subsystem
  Display{1..10,12} (11 alike) : Display
  Product2 : Product  Inputs=**  SaturateOnIntegerOverflow=on  OutDataTypeStr=Inherit: Same as first input
  enthalpy_MAPS : Subsystem
  thermo_turbine : Subsystem
  (DH)th/Tt4 : Outport
  S45 : Outport  Port=2
  Pt45 : Outport  Port=3
  Ht45 : Outport  Port=4
  Cp45 : Outport  Port=5
  F\A : Outport  Port=6
  Tt45 : Outport  Port=7
  wires:
  F/A/1 -> thermo_turbine/5(F/A), Product2/1
  S4/1 -> thermo_turbine/6(S4)
  " \"F/At= 0.9 * F/Acch\""/1 -> Product2/2
  Cp4/1 -> thermo_turbine/4(Cp4)
  Pt4/1 -> thermo_turbine/3(Pt4)
  enthalpy_MAPS/2((DH/T)th) -> (DH)th/Tt4/1
  Ht4/1 -> enthalpy_MAPS/1(Ht4)
  Tt4/1 -> enthalpy_MAPS/2(Tt4)
  Tt2.5/1 -> enthalpy_MAPS/3(Tt2.5)
  Nch/1 -> enthalpy_MAPS/4(Nch)
  TFth/1 -> enthalpy_MAPS/5(TFth)
  Product2/1 -> " HP turbine"/3(F_A)
  thermo_turbine/1(Pt45) -> " HP turbine"/1(Pt45), Display12/1, Pt45/1
  Wg4/1 -> " HP turbine"/5(Wg4)
  Wg45/1 -> " HP turbine"/6(Wg45)
  wach/1 -> " HP turbine"/7(wach)
  thermo_turbine/4(Cp45) -> " HP turbine"/2(Cp45_old), Display3/1
  Ht3/1 -> " HP turbine"/8(Ht3)
  " HP turbine"/2(Tt45) -> Tt45/1, Display9/1
  " HP turbine"/3(S45) -> Display8/1, S45/1
  " HP turbine"/4(Ht45) -> Display7/1, Ht45/1
  thermo_turbine/2(Tt45) -> Display1/1
  thermo_turbine/3(S45) -> Display2/1
  " HP turbine"/1(Cp45) -> Cp45/1, Display5/1
  " HP turbine"/5(F/A) -> Display6/1, F\A/1
  enthalpy_MAPS/1(Ht45s) -> thermo_turbine/1(Ht45s)
  enthalpy_MAPS/3(Ht45_old) -> Display10/1, " HP turbine"/4(Ht45_old), thermo_turbine/2(Ht45_old)

== system EngineModel_scaled_15_7_2016_with_new_maps/Double spool TFE CF6-50 steady state modeling (BOING 747-200)/Off- Design Module/LPC ==
  Tt13 : Inport
  Pt13 : Inport  Port=2
  Ht13 : Inport  Port=3
  S13 : Inport  Port=4
  Ncl : Inport  Port=5
  Zcl : Inport  Port=6
  (Po)Ref : Constant  Value=101325
  (To)Ref : Constant  Value=288
  Adiabatic compression : Subsystem
  Display{,1..5} (6 alike) : Display
  LPC Map : Subsystem
  Product1 : Product  Inputs=/*  SaturateOnIntegerOverflow=on  OutDataTypeStr=Inherit: Same as first input
  Product2 : Product  Inputs=*/  SaturateOnIntegerOverflow=on  OutDataTypeStr=Inherit: Same as first input
  Product3 : Product  Inputs=**  SaturateOnIntegerOverflow=on  OutDataTypeStr=Inherit: Same as first input
  Product4 : Product  Inputs=*/  SaturateOnIntegerOverflow=on  OutDataTypeStr=Inherit: Same as first input
  Sqrt : Sqrt  SaturateOnIntegerOverflow=on
  Tt2.5 : Outport
  Pt2.5 : Outport  Port=2
  Ht2.5 : Outport  Port=3
  S25 : Outport  Port=4
  Wacl : Outport  Port=5
  wires:
  Zcl/1 -> LPC Map/1(Zcl)
  Ncl/1 -> LPC Map/2(Ncf)
  Tt13/1 -> Adiabatic compression/1(Tt13), Product4/1
  Pt13/1 -> Adiabatic compression/2(Pt13), Product2/1
  LPC Map/2(etacl) -> Adiabatic compression/4(etacl)
  Product3/1 -> Product1/2
  Sqrt/1 -> Product1/1
  (Po)Ref/1 -> Product2/2
  LPC Map/3(MFPcl) -> Display5/1, Product3/2
  Product2/1 -> Product3/1
  (To)Ref/1 -> Product4/2
  Product4/1 -> Sqrt/1
  Product1/1 -> Display4/1, Wacl/1
  Adiabatic compression/1(Tt25) -> Display1/1, Tt2.5/1
  Adiabatic compression/2(Pt25) -> Display2/1, Pt2.5/1
  Adiabatic compression/3(Ht25) -> Display/1, Ht2.5/1
  LPC Map/1(Prcl) -> Adiabatic compression/3(Prcl)
  Ht13/1 -> Adiabatic compression/5(Ht13)
  S13/1 -> Adiabatic compression/6(S13)
  Adiabatic compression/4(S25) -> Display3/1, S25/1

== system EngineModel_scaled_15_7_2016_with_new_maps/Double spool TFE CF6-50 steady state modeling (BOING 747-200)/Off- Design Module/LPT ==
  Tt2 : Inport
  S45 : Inport  Port=2
  Pt45 : Inport  Port=3
  Ht45 : Inport  Port=4
  Cp45 : Inport  Port=5
  F/A : Inport  Port=6
  Tt45 : Inport  Port=7
  Ncf : Inport  Port=8
  TFtl : Inport  Port=9
  Display{1..3,10,12} (5 alike) : Display
  enthalpy_MAPS : Subsystem
  thermo_turbine : Subsystem
  (DH)th/Tt45 : Outport
  Pt5 : Outport  Port=2
  Ht5 : Outport  Port=3
  Tt5 : Outport  Port=4
  Mw5 : Outport  Port=5
  wires:
  S45/1 -> thermo_turbine/6(S45)
  Cp45/1 -> thermo_turbine/4(Cp45)
  Pt45/1 -> thermo_turbine/3(Pt45)
  enthalpy_MAPS/2((DH/T)tl) -> (DH)th/Tt45/1
  Ht45/1 -> enthalpy_MAPS/1(Ht45)
  Tt45/1 -> enthalpy_MAPS/2(Tt45)
  Tt2/1 -> enthalpy_MAPS/3(Tt2)
  Ncf/1 -> enthalpy_MAPS/4(Ncf)
  TFtl/1 -> enthalpy_MAPS/5(TFtl)
  F/A/1 -> thermo_turbine/5(F/A)
  thermo_turbine/1(Pt5) -> Display12/1, Pt5/1
  thermo_turbine/4(Cp5) -> Display3/1
  thermo_turbine/2(Tt5) -> Display1/1, Tt5/1
  thermo_turbine/3(S5) -> Display2/1
  enthalpy_MAPS/1(Ht5s) -> thermo_turbine/1(Ht5s)
  enthalpy_MAPS/3(Ht5) -> thermo_turbine/2(Ht5), Display10/1, Ht5/1
  thermo_turbine/6(Mw5) -> Mw5/1

== system EngineModel_scaled_15_7_2016_with_new_maps/Double spool TFE CF6-50 steady state modeling (BOING 747-200)/Off- Design Module/Ram ==
  Mo : Inport
  To : Inport  Port=2
  Po : Inport  Port=3
  Constant1 : Constant
  Constant2 : Constant  Value=0.2
  Constant3 : Constant  Value=3.5
  Display{,1..7} (8 alike) : Display
  If condition PRF : Subsystem
  Math Function1 : Math  Operator=pow  SignedPower=on  SaturateOnIntegerOverflow=on
  Math Function3 : Math  Operator=square  SignedPower=on  SaturateOnIntegerOverflow=on
  Product1 : Product
  Product2 : Product  Inputs=3
  Product7 : Product
  Ram compression : Subsystem
  add : Sum
  Tt2 : Outport
  Pt2 : Outport  Port=2
  Ht2 : Outport  Port=3
  S2 : Outport  Port=4
  wires:
  Mo/1 -> Math Function3/1, If condition PRF/1(Mo)
  Math Function3/1 -> Product7/1
  Constant2/1 -> Product7/2
  Product7/1 -> add/1
  Constant1/1 -> add/2
  add/1 -> Math Function1/1, Product1/1
  Constant3/1 -> Math Function1/2
  If condition PRF/1(etar) -> Product2/1, Display/1
  Math Function1/1 -> Product2/2
  Po/1 -> Display6/1, Product2/3
  ? -> ?
  To/1 -> Display5/1, Product1/2
  Product2/1 -> Pt2/1, Ram compression/2(Pt2), Display4/1
  Ram compression/1(Ht2) -> Ht2/1, Display2/1
  Ram compression/2(S2) -> S2/1, Display7/1
  Ram compression/3(Cp2) -> Display3/1
  Product1/1 -> Tt2/1, Display1/1, Ram compression/1(Tt2)

== system EngineModel_scaled_15_7_2016_with_new_maps/Double spool TFE CF6-50 steady state modeling (BOING 747-200)/solver/ LU Inverse ==
  A : Inport
  Identity Matrix : dspmtrx3/Identity Matrix  Inherit=on  N=5  Ts=1  dataType=double  isSigned=on  wordLen=16  udDataType=sfix(16)  fracBitsMode=Best precision  numFracBits=15  OutDataTypeStr=double  LastOutDataTypeStr=double
  LU Solver : Subsystem  AncestorBlock=dspsolvers/LU Solver  mask(LU Solver){}
      mask help: dsp:dspsolvers:LUSolver_MD
      mask init:
      | x=[ 0.135 .475 0.475 0.135 .135 NaN 0.55 0.64 0.64 0.55 0.55 NaN 0.685 0.73 NaN 0.685 0.73 NaN 0.775 0.865 0.865 0.775 0.775 ];
      | y=[ 0.2 0.2 0.7 0.7 0.2 NaN 0.2 0.2 0.7 0.7 0.2 NaN 0.4 0.4 NaN 0.45 0.45 NaN 0.2 0.2 0.7 0.7 0.2 ];
      mask Help: eval('blocksethelp');
      mask Display:
      | plot(x,y+0.05);
      | 
      | text(0.25,0.9,'AX=B (LU)');
      | 
      | text(0.12,0.15,'[m x m]');
  inv(A) : Outport
  wires:
  Identity Matrix/1 -> LU Solver/2(B)
  A/1 -> LU Solver/1(A), Identity Matrix/1
  LU Solver/1(X) -> inv(A)/1

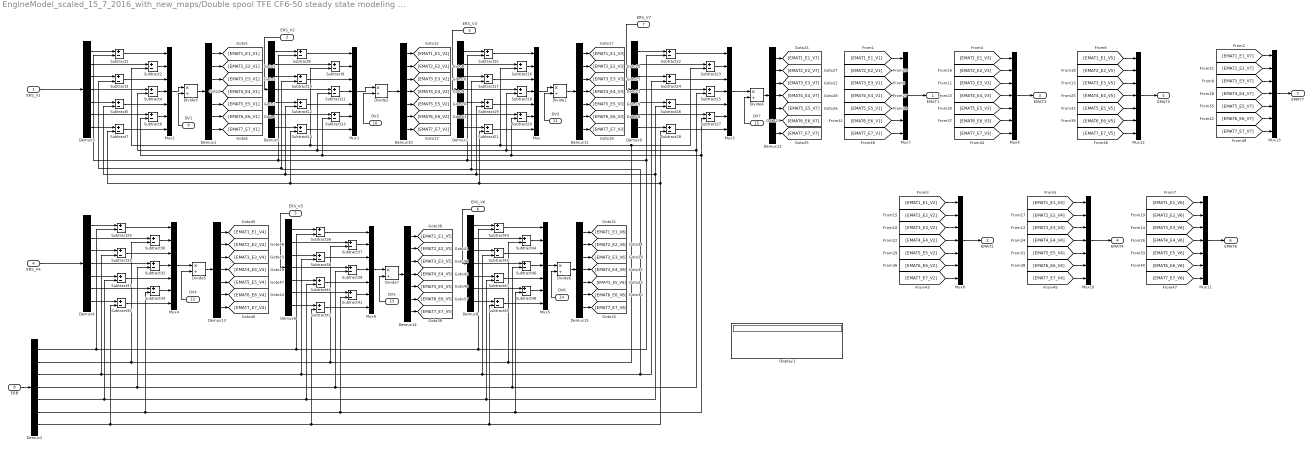
== system EngineModel_scaled_15_7_2016_with_new_maps/Double spool TFE CF6-50 steady state modeling (BOING 747-200)/solver/EMAT New ==
  ERS_V1 : Inport
  ERS_V2 : Inport  Port=2
  ERS_V3 : Inport  Port=3
  ERS_V4 : Inport  Port=4
  ERS_V5 : Inport  Port=5
  ERS_V6 : Inport  Port=6
  ERS_V7 : Inport  Port=7
  ERB : Inport  Port=8
  DV1 : Inport  Port=9
  DV2 : Inport  Port=10
  DV3 : Inport  Port=11
  DV4 : Inport  Port=12
  DV5 : Inport  Port=13
  DV6 : Inport  Port=14
  DV7 : Inport  Port=15
  Demux{1..15} (15 alike) : Demux  Outputs=7
  Display1 : Display
  Divide{1..7} (7 alike) : Product  Inputs=*/
  Mux{,1..13} (14 alike) : Mux  Inputs=7
  Subtract{1..49} (49 alike) : Sum  Inputs=+-
  EMAT1 : Outport
  EMAT2 : Outport  Port=2
  EMAT3 : Outport  Port=3
  EMAT4 : Outport  Port=4
  EMAT5 : Outport  Port=5
  EMAT6 : Outport  Port=6
  EMAT7 : Outport  Port=7
  wires:
  ERS_V6/1 -> Demux8/1
  ERS_V1/1 -> Demux3/1
  ERS_V7/1 -> Demux9/1
  ERB/1 -> Demux2/1
  Demux3/1 -> Subtract1/1
  Demux3/2 -> Subtract2/1
  Demux3/3 -> Subtract3/1
  Demux3/4 -> Subtract4/1
  Demux3/5 -> Subtract5/1
  Demux3/6 -> Subtract6/1
  Demux3/7 -> Subtract7/1
  Demux5/1 -> Subtract8/1
  Demux5/2 -> Subtract9/1
  Demux5/3 -> Subtract10/1
  Demux5/4 -> Subtract11/1
  Demux5/5 -> Subtract12/1
  Demux5/6 -> Subtract13/1
  Demux5/7 -> Subtract14/1
  Demux7/1 -> Subtract15/1
  Demux7/2 -> Subtract16/1
  Demux7/3 -> Subtract17/1
  Demux7/4 -> Subtract18/1
  Demux7/5 -> Subtract19/1
  Demux7/6 -> Subtract20/1
  Demux7/7 -> Subtract21/1
  Demux9/1 -> Subtract22/1
  Demux9/2 -> Subtract23/1
  Demux9/3 -> Subtract24/1
  Demux9/4 -> Subtract25/1
  Demux9/5 -> Subtract26/1
  Demux9/6 -> Subtract27/1
  Demux9/7 -> Subtract28/1
  Demux4/1 -> Subtract29/1
  Demux4/2 -> Subtract30/1
  Demux4/3 -> Subtract31/1
  Demux4/4 -> Subtract32/1
  Demux4/5 -> Subtract33/1
  Demux4/6 -> Subtract34/1
  Demux4/7 -> Subtract35/1
  Demux6/1 -> Subtract36/1
  Demux6/2 -> Subtract37/1
  Demux6/3 -> Subtract38/1
  Demux6/4 -> Subtract39/1
  Demux6/5 -> Subtract40/1
  Demux6/6 -> Subtract41/1
  Demux6/7 -> Subtract42/1
  Demux8/1 -> Subtract43/1
  Demux8/2 -> Subtract44/1
  Demux8/3 -> Subtract45/1
  Demux8/4 -> Subtract46/1
  Demux8/5 -> Subtract47/1
  Demux8/6 -> Subtract48/1
  Demux8/7 -> Subtract49/1
  Demux2/7 -> Subtract42/2, Subtract49/2, Subtract21/2, Subtract7/2, Subtract14/2, Subtract28/2, Subtract35/2
  Demux2/5 -> Subtract40/2, Subtract47/2, Subtract5/2, Subtract12/2, Subtract19/2, Subtract26/2, Subtract33/2
  Demux2/4 -> Subtract32/2, Subtract39/2, Subtract46/2, Subtract25/2, Subtract11/2, Subtract4/2, Subtract18/2
  Demux2/3 -> Subtract31/2, Subtract38/2, Subtract45/2, Subtract17/2, Subtract10/2, Subtract3/2, Subtract24/2
  Demux2/2 -> Subtract30/2, Subtract37/2, Subtract44/2, Subtract9/2, Subtract2/2, Subtract16/2, Subtract23/2
  Demux2/1 -> Subtract29/2, Subtract36/2, Subtract43/2, Subtract1/2, Subtract8/2, Subtract15/2, Subtract22/2
  Demux2/6 -> Subtract41/2, Subtract48/2, Subtract27/2, Subtract13/2, Subtract6/2, Subtract20/2, Subtract34/2
  Subtract15/1 -> Mux/1
  Subtract16/1 -> Mux/2
  Subtract17/1 -> Mux/3
  Subtract18/1 -> Mux/4
  Subtract19/1 -> Mux/5
  Subtract20/1 -> Mux/6
  Subtract21/1 -> Mux/7
  Mux/1 -> Divide1/1
  Mux1/1 -> Divide2/1
  Subtract8/1 -> Mux1/1
  Subtract9/1 -> Mux1/2
  Subtract10/1 -> Mux1/3
  Subtract11/1 -> Mux1/4
  Subtract12/1 -> Mux1/5
  Subtract13/1 -> Mux1/6
  Subtract14/1 -> Mux1/7
  Mux2/1 -> Divide3/1
  Subtract1/1 -> Mux2/1
  Subtract2/1 -> Mux2/2
  Subtract3/1 -> Mux2/3
  Subtract4/1 -> Mux2/4
  Subtract5/1 -> Mux2/5
  Subtract6/1 -> Mux2/6
  Subtract7/1 -> Mux2/7
  Mux3/1 -> Divide4/1
  Subtract22/1 -> Mux3/1
  Subtract23/1 -> Mux3/2
  Subtract24/1 -> Mux3/3
  Subtract25/1 -> Mux3/4
  Subtract26/1 -> Mux3/5
  Subtract27/1 -> Mux3/6
  Subtract28/1 -> Mux3/7
  Mux4/1 -> Divide5/1
  Subtract29/1 -> Mux4/1
  Subtract30/1 -> Mux4/2
  Subtract31/1 -> Mux4/3
  Subtract32/1 -> Mux4/4
  Subtract33/1 -> Mux4/5
  Subtract34/1 -> Mux4/6
  Subtract35/1 -> Mux4/7
  Mux5/1 -> Divide6/1
  Subtract43/1 -> Mux5/1
  Subtract44/1 -> Mux5/2
  Subtract45/1 -> Mux5/3
  Subtract46/1 -> Mux5/4
  Subtract47/1 -> Mux5/5
  Subtract48/1 -> Mux5/6
  Subtract49/1 -> Mux5/7
  Mux6/1 -> Divide7/1
  Subtract36/1 -> Mux6/1
  Subtract37/1 -> Mux6/2
  Subtract38/1 -> Mux6/3
  Subtract39/1 -> Mux6/4
  Subtract40/1 -> Mux6/5
  Subtract41/1 -> Mux6/6
  Subtract42/1 -> Mux6/7
  DV1/1 -> Divide3/2
  DV2/1 -> Divide2/2
  DV3/1 -> Divide1/2
  DV4/1 -> Divide5/2
  DV5/1 -> Divide7/2
  DV6/1 -> Divide6/2
  DV7/1 -> Divide4/2
  ERS_V2/1 -> Demux5/1
  ERS_V3/1 -> Demux7/1
  ERS_V4/1 -> Demux4/1
  ERS_V5/1 -> Demux6/1
  Divide3/1 -> Demux1/1
  Mux7/1 -> EMAT1/1
  Mux8/1 -> EMAT2/1
  Mux9/1 -> EMAT3/1
  Mux10/1 -> EMAT4/1
  Mux12/1 -> EMAT5/1
  Mux11/1 -> EMAT6/1
  Mux13/1 -> EMAT7/1
  Divide2/1 -> Demux10/1
  Divide1/1 -> Demux11/1
  Divide4/1 -> Demux12/1
  Divide5/1 -> Demux13/1
  Divide7/1 -> Demux14/1
  Divide6/1 -> Demux15/1
  Demux1/1 -> [EMAT1_E1_V1]
  Demux1/2 -> [EMAT2_E2_V1]
  Demux1/3 -> [EMAT3_E3_V1]
  Demux1/4 -> [EMAT4_E4_V1]
  Demux1/5 -> [EMAT5_E5_V1]
  Demux1/6 -> [EMAT6_E6_V1]
  Demux1/7 -> [EMAT7_E7_V1]
  Demux10/1 -> [EMAT1_E1_V2]
  Demux10/2 -> [EMAT2_E2_V2]
  Demux10/3 -> [EMAT3_E3_V2]
  Demux10/4 -> [EMAT4_E4_V2]
  Demux10/5 -> [EMAT5_E5_V2]
  Demux10/6 -> [EMAT6_E6_V2]
  Demux10/7 -> [EMAT7_E7_V2]
  Demux11/1 -> [EMAT1_E1_V3]
  Demux11/2 -> [EMAT2_E2_V3]
  Demux11/3 -> [EMAT3_E3_V3]
  Demux11/4 -> [EMAT4_E4_V3]
  Demux11/5 -> [EMAT5_E5_V3]
  Demux11/6 -> [EMAT6_E6_V3]
  Demux11/7 -> [EMAT7_E7_V3]
  Demux12/1 -> [EMAT1_E1_V7]
  Demux12/2 -> [EMAT2_E2_V7]
  Demux12/3 -> [EMAT3_E3_V7]
  Demux12/4 -> [EMAT4_E4_V7]
  Demux12/5 -> [EMAT5_E5_V7]
  Demux12/6 -> [EMAT6_E6_V7]
  Demux12/7 -> [EMAT7_E7_V7]
  Demux15/1 -> [EMAT1_E1_V6]
  Demux15/2 -> [EMAT2_E2_V6]
  Demux15/3 -> [EMAT3_E3_V6]
  Demux15/4 -> [EMAT4_E4_V6]
  Demux15/5 -> [EMAT5_E5_V6]
  Demux15/6 -> [EMAT6_E6_V6]
  Demux15/7 -> [EMAT7_E7_V6]
  Demux14/1 -> [EMAT1_E1_V5]
  Demux14/2 -> [EMAT2_E2_V5]
  Demux14/3 -> [EMAT3_E3_V5]
  Demux14/4 -> [EMAT4_E4_V5]
  Demux14/5 -> [EMAT5_E5_V5]
  Demux14/6 -> [EMAT6_E6_V5]
  Demux14/7 -> [EMAT7_E7_V5]
  Demux13/1 -> [EMAT1_E1_V4]
  Demux13/2 -> [EMAT2_E2_V4]
  Demux13/3 -> [EMAT3_E3_V4]
  Demux13/4 -> [EMAT4_E4_V4]
  Demux13/5 -> [EMAT5_E5_V4]
  Demux13/6 -> [EMAT6_E6_V4]
  Demux13/7 -> [EMAT7_E7_V4]
  [EMAT1_E1_V1] -> Mux7/1
  [EMAT2_E2_V1] -> Mux7/2
  [EMAT3_E3_V1] -> Mux7/3
  [EMAT4_E4_V1] -> Mux7/4
  [EMAT5_E5_V1] -> Mux7/5
  [EMAT6_E6_V1] -> Mux7/6
  [EMAT7_E7_V1] -> Mux7/7
  [EMAT7_E7_V2] -> Mux8/7
  [EMAT6_E6_V2] -> Mux8/6
  [EMAT5_E5_V2] -> Mux8/5
  [EMAT4_E4_V2] -> Mux8/4
  [EMAT3_E3_V2] -> Mux8/3
  [EMAT2_E2_V2] -> Mux8/2
  [EMAT1_E1_V2] -> Mux8/1
  [EMAT7_E7_V3] -> Mux9/7
  [EMAT6_E6_V3] -> Mux9/6
  [EMAT5_E5_V3] -> Mux9/5
  [EMAT4_E4_V3] -> Mux9/4
  [EMAT3_E3_V3] -> Mux9/3
  [EMAT2_E2_V3] -> Mux9/2
  [EMAT1_E1_V3] -> Mux9/1
  [EMAT7_E7_V4] -> Mux10/7
  [EMAT6_E6_V4] -> Mux10/6
  [EMAT5_E5_V4] -> Mux10/5
  [EMAT4_E4_V4] -> Mux10/4
  [EMAT3_E3_V4] -> Mux10/3
  [EMAT2_E2_V4] -> Mux10/2
  [EMAT1_E1_V4] -> Mux10/1
  [EMAT7_E7_V5] -> Mux12/7
  [EMAT6_E6_V5] -> Mux12/6
  [EMAT5_E5_V5] -> Mux12/5
  [EMAT4_E4_V5] -> Mux12/4
  [EMAT3_E3_V5] -> Mux12/3
  [EMAT2_E2_V5] -> Mux12/2
  [EMAT1_E1_V5] -> Mux12/1
  [EMAT1_E1_V6] -> Mux11/1
  [EMAT2_E2_V6] -> Mux11/2
  [EMAT3_E3_V6] -> Mux11/3
  [EMAT4_E4_V6] -> Mux11/4
  [EMAT5_E5_V6] -> Mux11/5
  [EMAT6_E6_V6] -> Mux11/6
  [EMAT7_E7_V6] -> Mux11/7
  [EMAT7_E7_V7] -> Mux13/7
  [EMAT6_E6_V7] -> Mux13/6
  [EMAT5_E5_V7] -> Mux13/5
  [EMAT4_E4_V7] -> Mux13/4
  [EMAT3_E3_V7] -> Mux13/3
  [EMAT2_E2_V7] -> Mux13/2
  [EMAT1_E1_V7] -> Mux13/1

== system EngineModel_scaled_15_7_2016_with_new_maps/Double spool TFE CF6-50 steady state modeling (BOING 747-200)/Error Due to Vs/Error Due To Dv1/COLD NOZZLE ==
  Pamb : Inport
  Tt13 : Inport  Port=2
  Ht13 : Inport  Port=3
  Mwa : Inport  Port=4
  Waf : Inport  Port=5
  Wacl : Inport  Port=6
  Demux : Demux  Outputs=6
      settings: DisplayOption=none
  Display : Display
  Display1 : Display
  Interpreted MATLAB Function : MATLABFcn  MATLABFcn=coldnozzle(u(1),u(2),u(3),u(4),u(5),u(6))  OutputDimensions=6
  Mux : Mux  Inputs=6
      settings: DisplayOption=signals
  A19 : Outport
  V19 : Outport  Port=2
  T19 : Outport  Port=3
  P19 : Outport  Port=4
  Pt19 : Outport  Port=5
  M19 : Outport  Port=6
  wires:
  Mux/1 -> Interpreted MATLAB Function/1
  Interpreted MATLAB Function/1 -> Demux/1
  Ht13/1 -> Mux/3
  Mwa/1 -> Mux/4
  Waf/1 -> Mux/5
  Wacl/1 -> Mux/6
  Demux/1 -> A19/1
  Demux/2 -> Display/1, V19/1
  Demux/3 -> Display1/1, T19/1
  Demux/4 -> P19/1
  Demux/5 -> Pt19/1
  Demux/6 -> M19/1
  Tt13/1 -> Mux/2
  Pamb/1 -> Mux/1

== system EngineModel_scaled_15_7_2016_with_new_maps/Double spool TFE CF6-50 steady state modeling (BOING 747-200)/Error Due to Vs/Error Due To Dv1/Combustor ==
  Tt3 : Inport
  Pt3 : Inport  Port=2
  Ht3 : Inport  Port=3
  Cp3 : Inport  Port=4
  Wach : Inport  Port=5
  Wf : Inport  Port=6
  (1-percent bleed airpcwb2) : Constant  Value=0.9
  Add1 : Sum
  Add2 : Sum
  Display{1..9,26} (10 alike) : Display
  Product : Product
  Thermo_combustor : Subsystem  TreatAsAtomicUnit=on
  combustor o/p enthalpy : Subsystem  TreatAsAtomicUnit=on
  combustor o/p pressure : Subsystem
  S4 : Outport
  Pt4 : Outport  Port=2
  Ht4 : Outport  Port=3
  Cp4 : Outport  Port=4
  F/A : Outport  Port=5
  Tt4 : Outport  Port=6
  wg4 : Outport  Port=7
  wg5 : Outport  Port=8
  wires:
  Pt3/1 -> combustor o/p pressure/1(Pt3)
  Tt3/1 -> combustor o/p pressure/2(Tt3)
  Wf/1 -> Add1/2, Add2/2, combustor o/p enthalpy/1("wf ")
  Ht3/1 -> combustor o/p enthalpy/3(Ht3)
  combustor o/p enthalpy/2(F_A) -> F/A/1, Thermo_combustor/4(F/A)
  Thermo_combustor/2(S4) -> Display7/1, S4/1
  Thermo_combustor/3(Cp4) -> Cp4/1
  Thermo_combustor/1(Tt4) -> Tt4/1, Display4/1
  Add1/1 -> Display2/1, wg5/1
  Wach/1 -> Product/2, combustor o/p pressure/3(wach), combustor o/p enthalpy/2(wach), Add1/1
  combustor o/p enthalpy/1(Ht4) -> Ht4/1, Display5/1, Thermo_combustor/3("Ht4 ")
  Product/1 -> Add2/1
  (1-percent bleed airpcwb2)/1 -> Product/1
  Add2/1 -> Display6/1, combustor o/p enthalpy/4(wg4), wg4/1
  Cp3/1 -> Thermo_combustor/2(Cp3)
  combustor o/p pressure/1(Pt4) -> Display1/1, Pt4/1, Thermo_combustor/1(Pt4)
  Thermo_combustor/4(Mw4) -> Display26/1
  Thermo_combustor/5(Rg) -> Display3/1
  Thermo_combustor/6(Gamma_g) -> Display8/1
  Thermo_combustor/7(a_g) -> Display9/1

== system EngineModel_scaled_15_7_2016_with_new_maps/Double spool TFE CF6-50 steady state modeling (BOING 747-200)/Error Due to Vs/Error Due To Dv1/E1 ==
  wacl : Inport
  wach : Inport  Port=2
  Display : Display
  Divide1 : Product  Inputs=*/
  Sum : Sum  Inputs=-+  SaturateOnIntegerOverflow=on
  E1 : Outport
  wires:
  wacl/1 -> Sum/1
  wach/1 -> Divide1/2, Sum/2
  Divide1/1 -> Display/1, E1/1
  Sum/1 -> Divide1/1

== system EngineModel_scaled_15_7_2016_with_new_maps/Double spool TFE CF6-50 steady state modeling (BOING 747-200)/Error Due to Vs/Error Due To Dv1/E2 ==
  Pt4 : Inport
  Tt4 : Inport  Port=2
  wg4 : Inport  Port=3
  TFth : Inport  Port=4
  Constant : Constant  Value=100000
  Display{,1..4} (5 alike) : Display
  Divide1 : Product  Inputs=/*
  Divide2 : Product  Inputs=/*
  Divide3 : Product  Inputs=/*
  Product5 : Product  Inputs=**  SaturateOnIntegerOverflow=on  OutDataTypeStr=Inherit: Same as first input
  Sqrt1 : Sqrt  SaturateOnIntegerOverflow=on
  Sum : Sum  Inputs=+-  SaturateOnIntegerOverflow=on
  E2 : Outport
  wires:
  Divide1/1 -> Display/1, E2/1
  Sum/1 -> Divide1/2
  TFth/1 -> Display1/1, Sum/2
  Divide2/1 -> Sum/1, Display2/1, Divide1/1
  Tt4/1 -> Sqrt1/1
  wg4/1 -> Display3/1, Product5/2
  Sqrt1/1 -> Product5/1
  Product5/1 -> Divide2/2
  Pt4/1 -> Divide3/2
  Constant/1 -> Divide3/1
  Divide3/1 -> Divide2/1, Display4/1

== system EngineModel_scaled_15_7_2016_with_new_maps/Double spool TFE CF6-50 steady state modeling (BOING 747-200)/Error Due to Vs/Error Due To Dv1/E3 ==
  Ht2.5 : Inport
  Ht3 : Inport  Port=2
  Wach : Inport  Port=3
  Wg4 : Inport  Port=4
  Tt4 : Inport  Port=5
  (DH)th/Tt4 : Inport  Port=6
  Constant : Constant  Value=4.184
  Display : Display
  Display1 : Display
  Divide1 : Product  Inputs=/*
  Divide2 : Product  Inputs=/*
  Divide3 : Product  Inputs=/*
  Product1 : Product  Inputs=**  SaturateOnIntegerOverflow=on  OutDataTypeStr=Inherit: Same as first input
  Product2 : Product  Inputs=**  SaturateOnIntegerOverflow=on  OutDataTypeStr=Inherit: Same as first input
  Sum : Sum  Inputs=+-  SaturateOnIntegerOverflow=on
  Sum1 : Sum  Inputs=+-  SaturateOnIntegerOverflow=on
  E3 : Outport
  wires:
  Ht2.5/1 -> Sum/2
  Ht3/1 -> Sum/1
  Sum/1 -> Product1/2
  Wach/1 -> Product1/1
  Wg4/1 -> Product2/1
  Tt4/1 -> Product2/2
  Product2/1 -> Divide1/1
  Divide1/1 -> Sum1/1, Divide2/1, Display1/1
  Sum1/1 -> Divide2/2
  Divide2/1 -> E3/1, Display/1
  Product1/1 -> Divide3/2
  Divide3/1 -> Divide1/2
  Constant/1 -> Divide3/1
  (DH)th/Tt4/1 -> Sum1/2
